simulink model "TestaBlocosUteis2"  (R2020b)
settings: Solver=FixedStepDiscrete  StartTime=0.0  StopTime=Plano.Tempo(end)  FixedStep=1  RelTol=1e-3
InitFcn:
  | CarregaTabelas
  | Plano=readtable('PlanoExperimentos.xlsx');
  | FreqIni=Plano.Frequencia(1);
  | PChegadaIni=Plano.PMonAlvo(1);
  | PSucIni=Interpola(FreqIni,PChegadaIni,MatrizSimulador,8);
  | VazaoIni=Interpola(FreqIni,PChegadaIni,MatrizSimulador,3);
  | FreqAlvoIni=FreqIni+1;
  | PMonAlvoIni=PChegadaIni+1;
  | VazaoAlvoIni=Interpola(FreqAlvoIni,PMonAlvoIni*1.019716,MatrizSimulador,3);
undefined symbols (not defined in the file): BTP, Interpola, MatrizSimulador, MatrizSimuladorContas, TabelaIsometricas, UIni, XIni
settings Model: Creator=leize  LastModifiedBy=leize

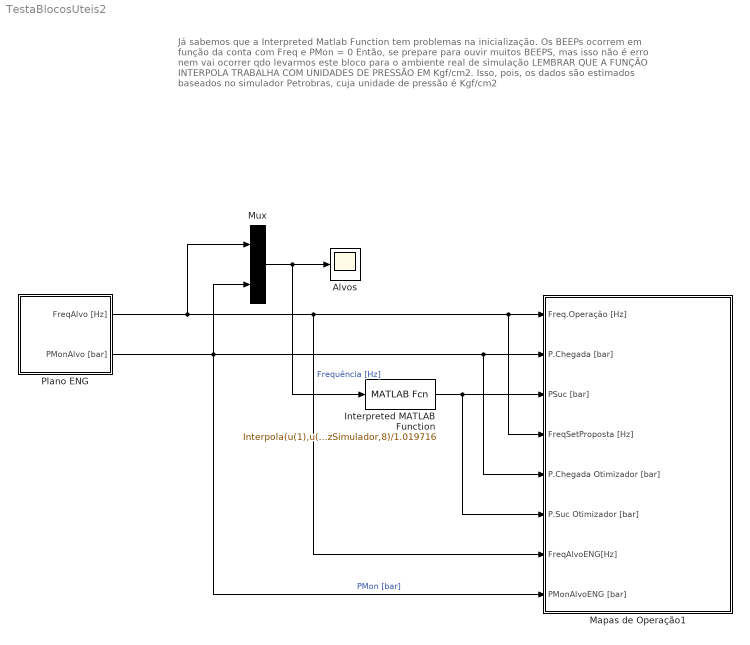
== system TestaBlocosUteis2 ==
  note: Já sabemos que a Interpreted Matlab Function tem problemas na inicialização.
      |
      | Os BEEPs ocorrem em função da conta com Freq e PMon = 0
      |
      | Então, se prepare para ouvir muitos BEEPS, mas isso não é erro nem vai ocorrer qdo levarmos este bloco para o ambiente real de simulação
      |
      | LEMBRAR QUE A FUNÇÃO INTERPOLA TRABALHA COM UNIDADES DE PRESSÃO EM Kgf/cm2. Isso, pois, os dados são estimados baseados no simulador Petrobras, cuja unidade de pressão é Kgf/cm2
  Alvos : Scope
  Interpreted MATLAB Function : MATLABFcn  MATLABFcn=Interpola(u(1),u(2)*1.019716,MatrizSimulador,8)/1.019716
  Mapas de Operação1 : Subsystem  mask{PlotaMapas=1, HabilitaRastro=1, Tsim=MatrizSimulador, TsimContas=MatrizSimuladorContas, BTP=BTP, TabelaIsometricas=TabelaIsometricas, FreqIni=UIni(1), PSucIni=XIni(1), PChegadaIni=XIni(2), FreqAlvoIni=FreqAlvoIni, PMonAlvoIni=PMonAlvoIni}
      mask prompts: PlotaMapas "Plotar Mapas (1/0)?"; HabilitaRastro "Habilita Rastro do Plot (1/0)?"; Tsim "Matriz do Simulador"; TsimContas "Matriz do Simulador para Limites"; BTP "Matriz BTP"; TabelaIsometricas "Tabela Curvas Isometricas"; FreqIni "Frequencia Inicial [Hz]"; PSucIni "Pressao de Succao Inicial [bar]"; PChegadaIni "PChegada Inicial [bar]"; FreqAlvoIni "Frequencia ALVO Inicial [Hz]"; PMonAlvoIni "PChegada ALVO [bar]"
      mask DialogControl DescTextVar Prompt: MAPAS DE OPERAÇÃO
      mask DialogControl ParameterGroupVar Prompt: Tabelas Petrobras e configurações dos Mapas de Operação
      mask DialogControl ParameterGroupVar_copy Prompt: Dados do Processo
      mask DialogControl ParameterGroupVar_copy_copy_copy Prompt: Dados Engenharia (Alvos)
  Mux : Mux  Inputs=2
  Plano ENG : Subsystem  mask{Plano=Plano}
      mask prompts: Plano "Plano de Execucao"
      mask DialogControl DescGroupVar Prompt: TABELA COM PLANO DE EXECUCAO
  wires:
  Mux/1 -> Alvos/1, Interpreted MATLAB Function/1
  Plano ENG/2(PMonAlvo [bar]) -> Mapas de Operação1/8(PMonAlvoENG [bar]), Mux/2, Mapas de Operação1/2(P.Chegada [bar]), Mapas de Operação1/5(P.Chegada Otimizador [bar])  "PMon [bar]"
  Plano ENG/1(FreqAlvo [Hz]) -> Mux/1, Mapas de Operação1/7(FreqAlvoENG[Hz]), Mapas de Operação1/4(FreqSetProposta [Hz]), Mapas de Operação1/1(Freq.Operação [Hz])  "Frequência [Hz]"
  Interpreted MATLAB Function/1 -> Mapas de Operação1/6(P.Suc Otimizador [bar]), Mapas de Operação1/3(PSuc [bar])

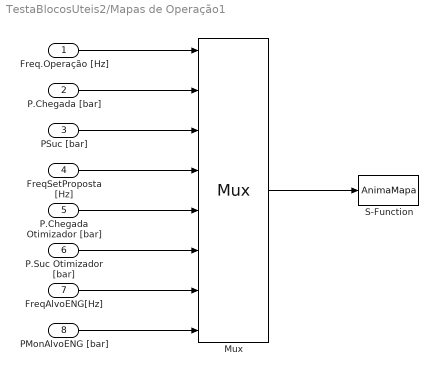
== system TestaBlocosUteis2/Mapas de Operação1 ==
  Freq.Operação [Hz] : Inport
  P.Chegada [bar] : Inport  Port=2
  PSuc [bar] : Inport  Port=3
  FreqSetProposta [Hz] : Inport  Port=4
  P.Chegada Otimizador [bar] : Inport  Port=5
  P.Suc Otimizador [bar] : Inport  Port=6
  FreqAlvoENG[Hz] : Inport  Port=7
  PMonAlvoENG [bar] : Inport  Port=8
  Mux : Mux  Inputs=8
  S-Function : S-Function  FunctionName=AnimaMapa  Parameters=PlotaMapas,Tsim,TsimContas,BTP,FreqIni, PChegadaIni,PSucIni,FreqAlvoIni,PMonAlvoIni,HabilitaRastro,TabelaIsometricas  SFunctionDeploymentMode=off  EnableBusSupport=off
  wires:
  Freq.Operação [Hz]/1 -> Mux/1
  Mux/1 -> S-Function/1
  P.Chegada [bar]/1 -> Mux/2
  PSuc [bar]/1 -> Mux/3
  P.Chegada Otimizador [bar]/1 -> Mux/5
  P.Suc Otimizador [bar]/1 -> Mux/6
  FreqAlvoENG[Hz]/1 -> Mux/7
  PMonAlvoENG [bar]/1 -> Mux/8
  FreqSetProposta [Hz]/1 -> Mux/4

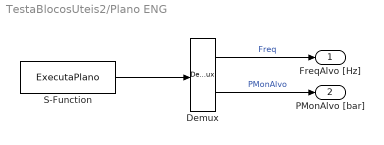
== system TestaBlocosUteis2/Plano ENG ==
  Demux : Demux  Outputs=2
  S-Function : S-Function  FunctionName=ExecutaPlano  Parameters=Plano  SFunctionDeploymentMode=off  EnableBusSupport=off
  FreqAlvo [Hz] : Outport
  PMonAlvo [bar] : Outport  Port=2
  wires:
  S-Function/1 -> Demux/1
  Demux/1 -> FreqAlvo [Hz]/1  "Freq"
  Demux/2 -> PMonAlvo [bar]/1  "PMonAlvo"
